simulink model "validate_engine_start_stop"  (R2015a)
settings: Solver=ode45  StartTime=0.0  StopTime=10.0  RelTol=1e-3
settings Model: Creator=Piyush  LastModifiedBy=Piyush

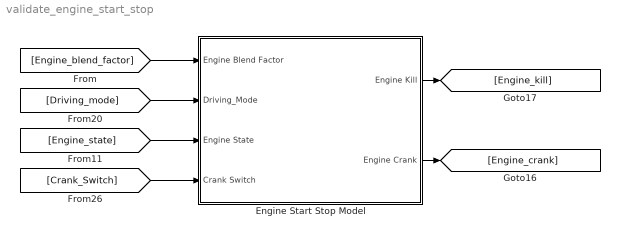
== system validate_engine_start_stop ==
  Engine Start Stop Model : Subsystem
  wires:
  [Engine_blend_factor] -> Engine Start Stop Model/1(Engine Blend Factor)
  [Engine_state] -> Engine Start Stop Model/3(Engine State)
  [Driving_mode] -> Engine Start Stop Model/2(Driving_Mode)
  [Crank_Switch] -> Engine Start Stop Model/4(Crank Switch)
  Engine Start Stop Model/2(Engine Crank) -> [Engine_crank]
  Engine Start Stop Model/1(Engine Kill) -> [Engine_kill]

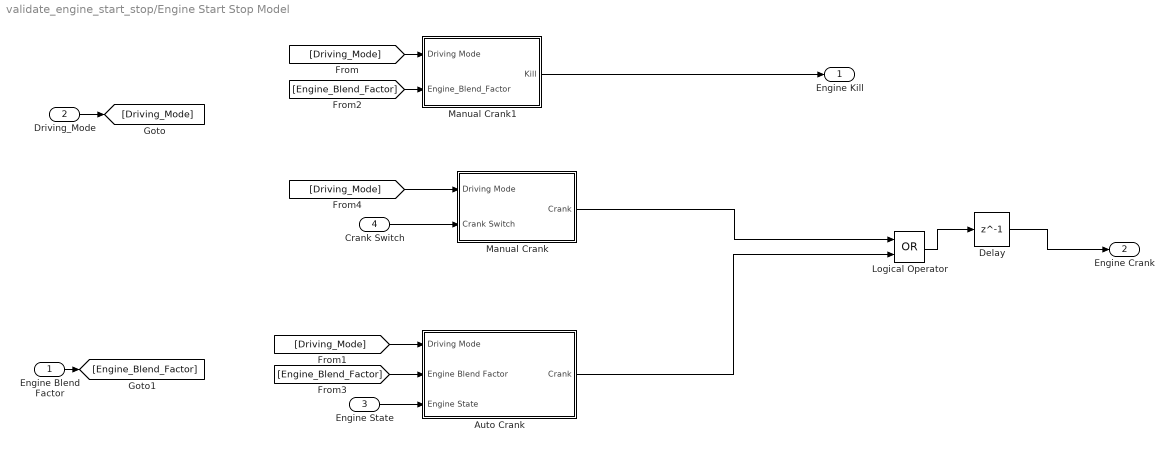
== system validate_engine_start_stop/Engine Start Stop Model ==
  Engine Blend Factor : Inport
  Driving_Mode : Inport  Port=2
  Engine State : Inport  Port=3
  Crank Switch : Inport  Port=4
  Auto Crank : Subsystem
  Delay : Delay  DelayLength=1  InitialCondition=0
  Logical Operator : Logic  Operator=OR  AllPortsSameDT=off  OutDataTypeStr=boolean
  Manual Crank : Subsystem
  Manual Crank1 : Subsystem
  Engine Kill : Outport
  Engine Crank : Outport  Port=2
  wires:
  Logical Operator/1 -> Delay/1
  Crank Switch/1 -> Manual Crank/2(Crank Switch)
  Engine State/1 -> Auto Crank/3(Engine State)
  Manual Crank1/1(Kill) -> Engine Kill/1
  Driving_Mode/1 -> [Driving_Mode]
  Engine Blend Factor/1 -> [Engine_Blend_Factor]
  [Driving_Mode] -> Manual Crank1/1(Driving Mode)
  [Driving_Mode] -> Auto Crank/1(Driving Mode)
  [Engine_Blend_Factor] -> Manual Crank1/2(Engine_Blend_Factor)
  [Engine_Blend_Factor] -> Auto Crank/2(Engine Blend Factor)
  [Driving_Mode] -> Manual Crank/1(Driving Mode)
  Auto Crank/1(Crank) -> Logical Operator/2
  Manual Crank/1(Crank) -> Logical Operator/1
  Delay/1 -> Engine Crank/1

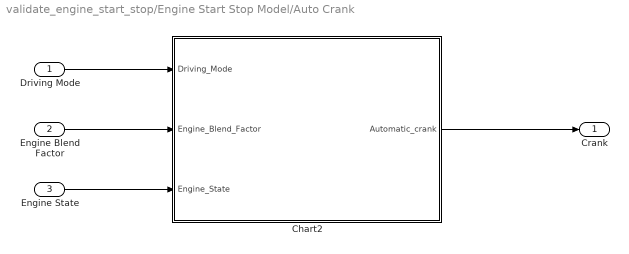
== system validate_engine_start_stop/Engine Start Stop Model/Auto Crank ==
  Driving Mode : Inport
  Engine Blend Factor : Inport  Port=2
  Engine State : Inport  Port=3
  Chart2 : Stateflow chart  TreatAsAtomicUnit=on
  Crank : Outport
  wires:
  Chart2/1(Automatic_crank) -> Crank/1
  Engine State/1 -> Chart2/3(Engine_State)
  Engine Blend Factor/1 -> Chart2/2(Engine_Blend_Factor)
  Driving Mode/1 -> Chart2/1(Driving_Mode)

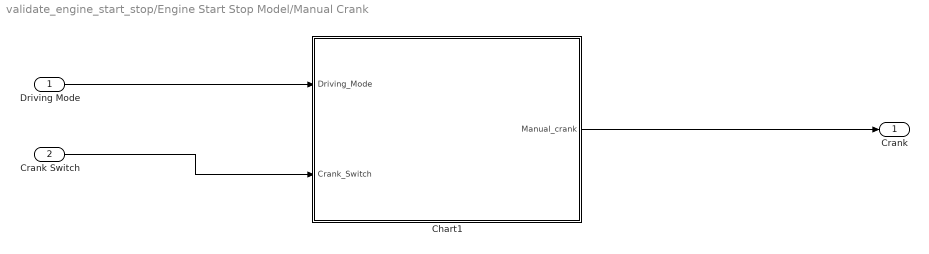
== system validate_engine_start_stop/Engine Start Stop Model/Manual Crank ==
  Driving Mode : Inport
  Crank Switch : Inport  Port=2
  Chart1 : Stateflow chart  TreatAsAtomicUnit=on
  Crank : Outport
  wires:
  Driving Mode/1 -> Chart1/1(Driving_Mode)
  Crank Switch/1 -> Chart1/2(Crank_Switch)
  Chart1/1(Manual_crank) -> Crank/1

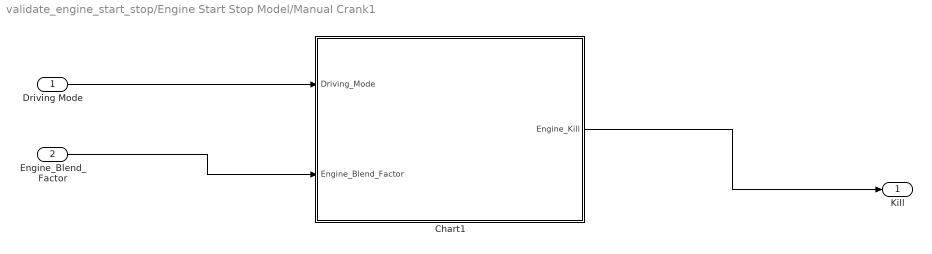
== system validate_engine_start_stop/Engine Start Stop Model/Manual Crank1 ==
  Driving Mode : Inport
  Engine_Blend_Factor : Inport  Port=2
  Chart1 : Stateflow chart  TreatAsAtomicUnit=on
  Kill : Outport
  wires:
  Engine_Blend_Factor/1 -> Chart1/2(Engine_Blend_Factor)
  Driving Mode/1 -> Chart1/1(Driving_Mode)
  Chart1/1(Engine_Kill) -> Kill/1

== stateflow chart validate_engine_start_stop/Engine Start Stop Model/Manual Crank/Chart1 ==
  state CRANK_ON
    during: Manual_crank=1;
  state CRANKOFF
    during: Manual_crank=0;
  CRANK_ON -> CRANKOFF : [Driving_Mode==1||Driving_Mode==2]
  CRANKOFF -> CRANK_ON : [Crank_Switch==1&&Driving_Mode==3]
  (default) -> CRANKOFF
  data: Driving_Mode input; Crank_Switch input; Manual_crank output

== stateflow chart validate_engine_start_stop/Engine Start Stop Model/Auto Crank/Chart2 ==
  state CRANK_ON
    during: Automatic_crank=1;
  state CRANKOFF
    during: Automatic_crank=0;
  CRANK_ON -> CRANKOFF [order 1] : [Driving_Mode==1||Driving_Mode==3]
  CRANK_ON -> CRANKOFF [order 2] : [Driving_Mode==2&&Engine_Blend_Factor<0.01]
  CRANKOFF -> CRANK_ON : [Driving_Mode==2&&Engine_Blend_Factor>0.01&&Engine_State==1]
  (default) -> CRANKOFF
  data: Driving_Mode input; Engine_Blend_Factor input; Automatic_crank output; Engine_State input

== stateflow chart validate_engine_start_stop/Engine Start Stop Model/Manual Crank1/Chart1 ==
  state KILL_ON
    during: Engine_Kill=1;
  state KILL_OFF
    during: Engine_Kill=0;
  KILL_ON -> KILL_OFF [order 2] : [Driving_Mode==2&&Engine_Blend_Factor>0.01]
  KILL_ON -> KILL_OFF [order 1] : [Driving_Mode==3]
  KILL_OFF -> KILL_ON [order 1] : [Driving_Mode==1]
  KILL_OFF -> KILL_ON [order 2] : [Driving_Mode==2&&Engine_Blend_Factor<0.01]
  (default) -> KILL_OFF
  data: Driving_Mode input; Engine_Blend_Factor input; Engine_Kill output
